simulink model "udp_tracker"  (R2024b)
settings: Solver=VariableStepAuto  StartTime=0.0  StopTime=100.0  RelTol=1e-3
undefined symbols (not defined in the file): f
libraries: instrumentlib x1
settings Model: Creator=PC  LastModifiedBy=PC

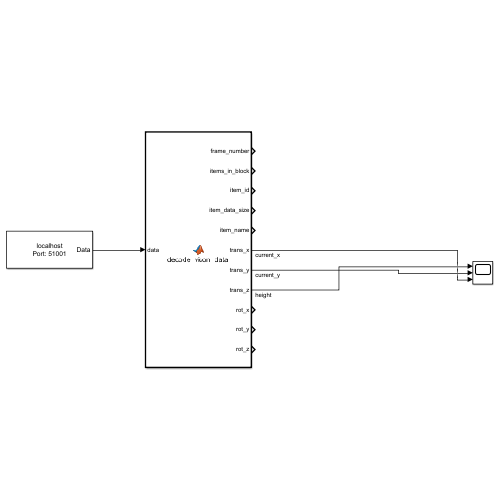
[thumbnail: Simulink's stored preview of the top-level diagram]
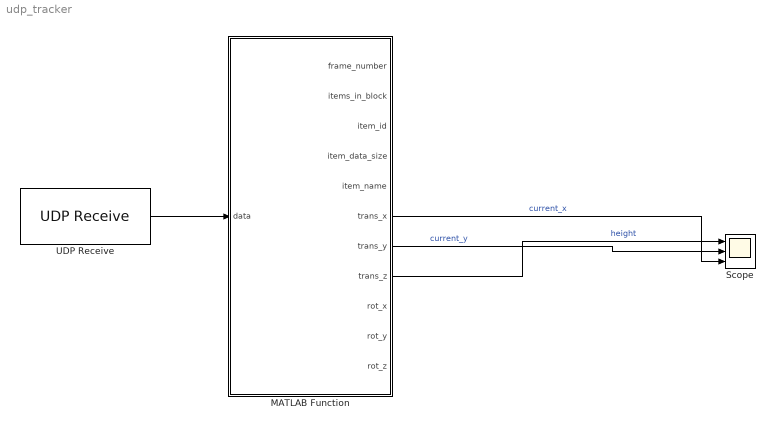
== system udp_tracker ==
  MATLAB Function : MATLAB Function  TreatAsAtomicUnit=on
  Scope : Scope  NumInputPorts=3
  UDP Receive : instrumentlib/UDP Receive  LocalAddress=localhost  LocalPort=51001  EnablePortSharing=off  Host=localhost  Port=9090  GetLatestData=on  DataSize=[1024, 1]  DataType=uint8  ASCIIFormatting=%f,  Terminator=LF  CustomTerminator=10  ByteOrder=big-endian  EnableBlockingMode=on  Timeout=10  SampleTime=0.02  SimulateUsing=Interpreted execution
  wires:
  UDP Receive/1 -> MATLAB Function/1(data)
  MATLAB Function/8(trans_z) -> Scope/1  "height"
  MATLAB Function/7(trans_y) -> Scope/2  "current_y"
  MATLAB Function/6(trans_x) -> Scope/3  "current_x"

== matlab function udp_tracker/MATLAB Function ==
  data: data input; frame_number output; items_in_block output; item_id output; item_data_size output; item_name output; trans_x output; trans_y output; trans_z output; rot_x output; rot_y output; rot_z output
function [frame_number, items_in_block, item_id, item_data_size, item_name, ...
    trans_x, trans_y, trans_z, rot_x, rot_y, rot_z] = decode_vicon_data(data)
    % Define expected output sizes explicitly
    % Set up each output as an array with dimensions (1x1) or (8x1) as needed.

    % Initialize output arrays
    frame_number = zeros(1, 1, 'uint32');  % Explicitly scalar output
    items_in_block = zeros(1, 1, 'uint8');  % Explicitly scalar output
    item_id = zeros(1, 1, 'uint8');        % Explicitly scalar output
    item_data_size = zeros(1, 1, 'uint16'); % Explicitly scalar output
    item_name = zeros(24, 1, 'uint8');     % 24 bytes for item name, uint8 array
    trans_x = zeros(1, 1, 'double');       % Scalar, double
    trans_y = zeros(1, 1, 'double');       % Scalar, double
    trans_z = zeros(1, 1, 'double');       % Scalar, double
    rot_x = zeros(1, 1, 'double');         % Scalar, double
    rot_y = zeros(1, 1, 'double');         % Scalar, double
    rot_z = zeros(1, 1, 'double');         % Scalar, double

    % Frame Number (4 bytes, uint32), scalar
    frame_number = typecast(data(1:4), 'uint32');
    
    % ItemsInBlock (1 byte, uint8)
    items_in_block = uint8(data(5));  % Scalar uint8
    
    % Item ID (1 byte, uint8) (0 for object data)
    item_id = uint8(data(6));  % Scalar uint8
    
    % Item Data Size (2 bytes, uint16)
    item_data_size = typecast(data(7:8), 'uint16');  % Scalar uint16
    
    % Item Name (24 bytes, uint8) converted from char
    item_name = uint8(data(9:32));  % Cast to uint8 (ASCII values of characters)
    
    % Translation (TransX, TransY, TransZ) - 8 bytes each (double)
    trans_x = typecast(data(33:40), 'double');
    trans_y = typecast(data(41:48), 'double');
    trans_z = typecast(data(49:56), 'double');
    
    % Rotation (RotX, RotY, RotZ) - 8 bytes each (double)
    rot_x = typecast(data(57:64), 'double');
    rot_y = typecast(data(65:72), 'double');
    rot_z = typecast(data(73:80), 'double');
end
